simulink model "bh_wheel_dynamics_COMPARE_hand_SEME_to_MEME"  (R2019a)
settings: Solver=ode15s  StartTime=0.0  StopTime=80  FixedStep=0.001  RelTol=1e-6  EnableMultiTasking=on
undefined symbols (not defined in the file or in its folder): Ic_xx_val, sigbuilder_block
libraries: simulink_extras x6
settings Model: Creator=bhorton  LastModifiedBy=bhorton
settings SolverCC: ZeroCrossAlgorithm=Adaptive
settings DataIOCC: SaveOutput=off  SignalLogging=off  DSMLogging=off  VisualizeSimOutput=off  SaveTime=off  ReturnWorkspaceOutputs=off
settings OptimizationCC: LifeSpan=inf
settings DebuggingCC: AllowSymbolicDim=off  SFUnexpectedBacktrackingDiag=warning  SFNoUnconditionalDefaultTransitionDiag=warning  SFExecutionAtInitializationDiag=none  ArithmeticOperatorsInVariantConditions=warning
settings ModelReferenceCC: PropagateSignalLabelsOutOfModel=off
settings SFSimCC: SimUseLocalCustomCode=off
settings RTWCC: RTWUseLocalCustomCode=off
settings CodeAppCC: StateflowObjectComments=on
settings GRTTargetCC: TargetLangStandard=C89/C90 (ANSI)
settings ConfigComp: CovMetricSettings=dw  CovHtmlReporting=on  CovSaveCumulativeToWorkspaceVar=on  CovSaveSingleToWorkspaceVar=on  CovExternalEMLEnable=off
settings SimscapeCC: SimscapeNormalizeSystem=off

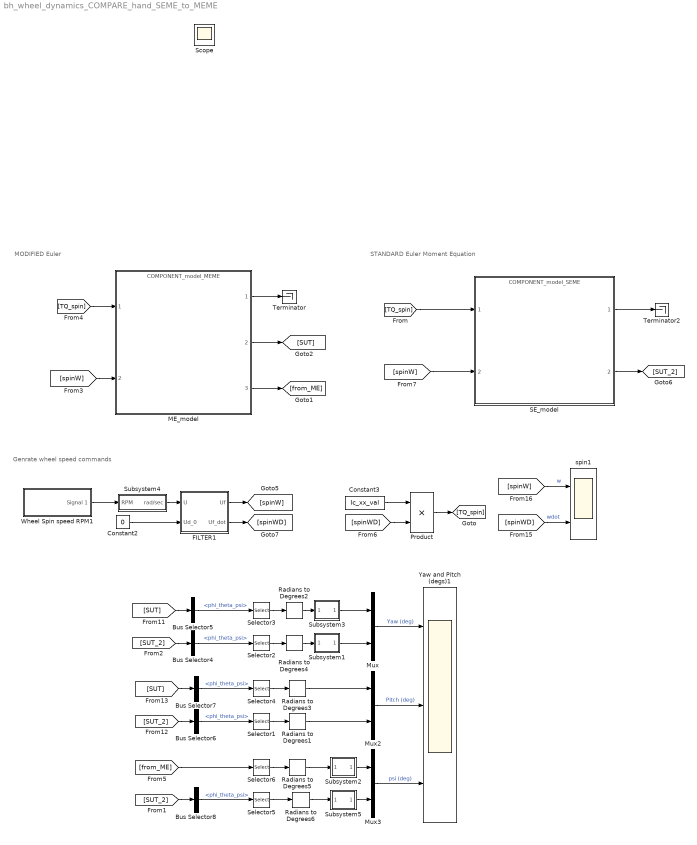
== system bh_wheel_dynamics_COMPARE_hand_SEME_to_MEME ==
  note: MODIFIED Euler
  note: STANDARD Euler Moment Equation
  note: Genrate wheel speed commands
  Bus Selector{4..8} (5 alike) : BusSelector  OutputSignals=phi_theta_psi
  Constant2 : Constant  Value=0
  Constant3 : Constant  Value=Ic_xx_val
  FILTER1 : Subsystem
  ME_model : ModelReference  ModelNameDialog=COMPONENT_model_MEME.slx  SimulationMode=Normal  ModelReferenceVersion=1.567
  Mux : Mux  Inputs=2
  Mux2 : Mux  Inputs=2
  Mux3 : Mux  Inputs=2
  Product : Product
  Radians to Degrees{1..6} (6 alike) : simulink_extras/Transformations/Radians to Degrees
  SE_model : ModelReference  ModelNameDialog=COMPONENT_model_SEME.slx  SimulationMode=Normal  ModelReferenceVersion=1.562
  Selector1 : Selector  InputPortWidth=3  IndexOptions=Index vector (dialog)  Indices=2  OutputSizes=1
  Selector2 : Selector  InputPortWidth=3  IndexOptions=Index vector (dialog)  Indices=1  OutputSizes=1
  Selector3 : Selector  InputPortWidth=3  IndexOptions=Index vector (dialog)  Indices=1  OutputSizes=1
  Selector4 : Selector  InputPortWidth=3  IndexOptions=Index vector (dialog)  Indices=2  OutputSizes=1
  Selector5 : Selector  InputPortWidth=3  IndexOptions=Index vector (dialog)  Indices=3  OutputSizes=1
  Selector6 : Selector  InputPortWidth=2  IndexOptions=Index vector (dialog)  Indices=2  OutputSizes=1
  Subsystem1 : Subsystem
      mask Display: disp(sprintf('Mod\n360'))
  Subsystem2 : Subsystem
      mask Display: disp(sprintf('Mod\n360'))
  Subsystem3 : Subsystem
      mask Display: disp(sprintf('Mod\n360'))
  Subsystem4 : Subsystem
  Subsystem5 : Subsystem
      mask Display: disp(sprintf('Mod\n360'))
  Terminator : Terminator
  Terminator2 : Terminator
  Wheel Spin speed RPM1 : Subsystem  Tag=STV Subsys  LoadFcn=sigbuilder_block('load');  StartFcn=sigbuilder_block('start');  StopFcn=sigbuilder_block('stop');  ClipboardFcn=sigbuilder_block('clipboard');  mask(Sigbuilder block){tuvar=[0:10]}
      mask help: Simulink:masks:SigbuilderBlock_MD
      mask init:
      | if ~strcmp(get_param(bdroot(gcbh),'SimulationStatus'),'stopped') tuvar = sigbuilder_block('maskInit'); end
      settings: CopyFcn=sigbuilder_block('copy');  DeleteFcn=sigbuilder_block('delete');  ModelCloseFcn=sigbuilder_block('modelClose');  PreSaveFcn=sigbuilder_block('preSave');  PauseFcn=sigbuilder_block('pause');  ContinueFcn=sigbuilder_block('continue');  NameChangeFcn=sigbuilder_block('namechange');  OpenFcn=sigbuilder_block('open',[6 6 1428 740.25 ]);  CloseFcn=sigbuilder_block('close');
      mask Display: plot(0, 0, 100, 100,[2, 2, 32, 32, 2], [68, 8, 8, 68, 68],[32, 2], [38, 38], [32, 19, 2],[53, 60, 44], [32, 17, 17, 2],[16, 16, 31, 31]);txt = getActiveGroup(gcbh);text(2, 100, txt,'verticalAlignment', 'top');
  Yaw and Pitch (degs)1 : Scope  NumInputPorts=3
  spin1 : Scope  NumInputPorts=2
  Scope : Scope
  wires:
  Selector1/1 -> Radians to Degrees1/1
  Radians to Degrees4/1 -> Subsystem1/1(In1)
  Radians to Degrees1/1 -> Mux2/2
  Selector2/1 -> Radians to Degrees4/1
  [SUT_2] -> Bus Selector6/1
  [SUT_2] -> Bus Selector4/1
  Bus Selector5/1 -> Selector3/1  "<phi_theta_psi>"
  Radians to Degrees2/1 -> Subsystem3/1(In1)
  Selector4/1 -> Radians to Degrees3/1
  Mux2/1 -> Yaw and Pitch (degs)1/2  "Pitch (deg)"
  Subsystem1/1(Out1) -> Mux/2
  [SUT] -> Bus Selector7/1
  Subsystem3/1(Out1) -> Mux/1
  Mux/1 -> Yaw and Pitch (degs)1/1  "Yaw (deg)"
  Bus Selector7/1 -> Selector4/1  "<phi_theta_psi>"
  Radians to Degrees3/1 -> Mux2/1
  Selector3/1 -> Radians to Degrees2/1
  Bus Selector6/1 -> Selector1/1  "<phi_theta_psi>"
  Bus Selector4/1 -> Selector2/1  "<phi_theta_psi>"
  [SUT] -> Bus Selector5/1
  Mux3/1 -> Yaw and Pitch (degs)1/3  "psi (deg)"
  [SUT_2] -> Bus Selector8/1
  Bus Selector8/1 -> Selector5/1  "<phi_theta_psi>"
  Selector5/1 -> Radians to Degrees6/1
  Selector6/1 -> Radians to Degrees5/1
  ME_model/2 -> [SUT]
  [TQ_spin] -> ME_model/1
  SE_model/2 -> [SUT_2]
  [spinW] -> SE_model/2
  [TQ_spin] -> SE_model/1
  SE_model/1 -> Terminator2/1
  ME_model/1 -> Terminator/1
  [spinW] -> ME_model/2
  FILTER1/2(Uf_dot) -> [spinWD]
  [spinWD] -> Product/2
  Wheel Spin speed RPM1/1(Signal 1) -> Subsystem4/1(RPM)
  Constant3/1 -> Product/1
  Constant2/1 -> FILTER1/2(Ud_0)
  FILTER1/1(Uf) -> [spinW]
  Subsystem4/1(rad/sec) -> FILTER1/1(U)
  [spinWD] -> spin1/2  "wdot"
  [spinW] -> spin1/1  "w"
  Product/1 -> [TQ_spin]
  ME_model/3 -> [from_ME]
  [from_ME] -> Selector6/1
  Radians to Degrees5/1 -> Subsystem2/1(In1)
  Radians to Degrees6/1 -> Subsystem5/1(In1)
  Subsystem2/1(Out1) -> Mux3/1
  Subsystem5/1(Out1) -> Mux3/2

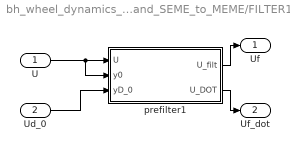
== system bh_wheel_dynamics_COMPARE_hand_SEME_to_MEME/FILTER1 ==
  U : Inport
  Ud_0 : Inport  Port=2
  prefilter1 : Subsystem  mask(Derivative Estimation){wn=2*pi*5, p=1}
      mask prompts: wn "Natural frequency, wn (rad/sec)"; p "Damping ratio, p"
      mask help:
      | A simple derivative estimator using a 2nd order representation between input and output.
      |
      | The integrators use a discrete FORWARd Euler rule, and a sample time needs to be specified.
      mask init:
      | str1 = sprintf('wn = %.2f', wn);
      | str2 = sprintf('p  = %.2f', p);
      | %str3 = sprintf('dt = %.2f', dt);
      | %str = char(str1,str2,str3);
      | %str3 = sprintf('dt = %.2f', dt);
      | str = char(str1,str2);
      mask Display: disp(str)
  Uf : Outport
  Uf_dot : Outport  Port=2
  wires:
  Ud_0/1 -> prefilter1/3(yD_0)
  prefilter1/2(U_DOT) -> Uf_dot/1
  prefilter1/1(U_filt) -> Uf/1
  U/1 -> prefilter1/2(y0), prefilter1/1(U)

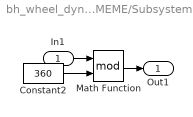
== system bh_wheel_dynamics_COMPARE_hand_SEME_to_MEME/Subsystem1 ==
  In1 : Inport
  Constant2 : Constant  Value=360
  Math Function : Math  Operator=mod  SaturateOnIntegerOverflow=on
  Out1 : Outport
  wires:
  Math Function/1 -> Out1/1
  In1/1 -> Math Function/1
  Constant2/1 -> Math Function/2

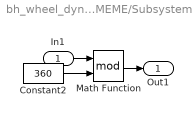
== system bh_wheel_dynamics_COMPARE_hand_SEME_to_MEME/Subsystem2 ==
  In1 : Inport
  Constant2 : Constant  Value=360
  Math Function : Math  Operator=mod  SaturateOnIntegerOverflow=on
  Out1 : Outport
  wires:
  Math Function/1 -> Out1/1
  In1/1 -> Math Function/1
  Constant2/1 -> Math Function/2

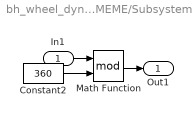
== system bh_wheel_dynamics_COMPARE_hand_SEME_to_MEME/Subsystem3 ==
  In1 : Inport
  Constant2 : Constant  Value=360
  Math Function : Math  Operator=mod  SaturateOnIntegerOverflow=on
  Out1 : Outport
  wires:
  Math Function/1 -> Out1/1
  In1/1 -> Math Function/1
  Constant2/1 -> Math Function/2

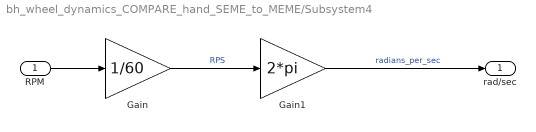
== system bh_wheel_dynamics_COMPARE_hand_SEME_to_MEME/Subsystem4 ==
  RPM : Inport
  Gain : Gain  Gain=1/60
  Gain1 : Gain  Gain=2*pi
  rad/sec : Outport
  wires:
  RPM/1 -> Gain/1
  Gain/1 -> Gain1/1  "RPS"
  Gain1/1 -> rad/sec/1  "radians_per_sec"

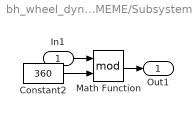
== system bh_wheel_dynamics_COMPARE_hand_SEME_to_MEME/Subsystem5 ==
  In1 : Inport
  Constant2 : Constant  Value=360
  Math Function : Math  Operator=mod  SaturateOnIntegerOverflow=on
  Out1 : Outport
  wires:
  Math Function/1 -> Out1/1
  In1/1 -> Math Function/1
  Constant2/1 -> Math Function/2

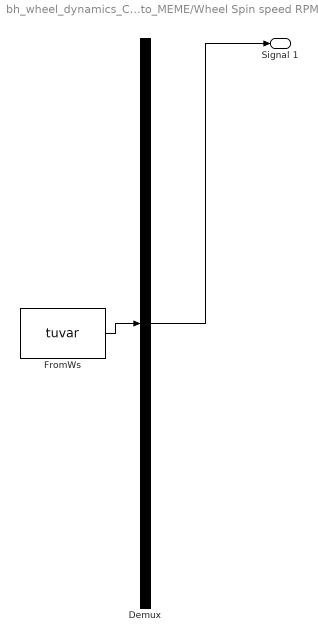
== system bh_wheel_dynamics_COMPARE_hand_SEME_to_MEME/Wheel Spin speed RPM1 ==
  Demux : Demux  Tag=STV Demux  Outputs=1
  FromWs : FromWorkspace  Tag=STV FromWs  VariableName=tuvar  SampleTime=0
      SigBuilderData=|
      | common.afterFinalStr = 'Extrapolate'
      | common.sampleTime = 0
      | dataSet(1).timeRange = [0 60]
      | dataSet(1).name = 'RAMP_DOWN'
      | dataSet(2).timeRange = [0 80]
      | dataSet(2).name = 'STAIRCASE_DOWN'
      | dataSet(3).timeRange = [0 60]
      | dataSet(3).name = 'STAIRCASE_UP'
      | sbobj.Groups(1).Name = 'RAMP_DOWN'
      | sbobj.Groups(1).Signals.Name = 'Signal 1'
      | sbobj.Groups(1).Signals.XData = [0 60]
      | sbobj.Groups(1).Signals.YData = [2000 0]
      | sbobj.Groups(1).TimeRange = [0 60]
      | sbobj.Groups(2).Name = 'STAIRCASE_DOWN'
      | sbobj.Groups(2).Signals.Name = 'Signal 1'
      | sbobj.Groups(2).Signals.XData = [0 10.1 10.1 20 20 30 30 39.9 39.9 49.9 49.9 60.2 60.2 70 70 80]
      | sbobj.Groups(2).Signals.YData = [2000 2000 1500 1500 1000 1000 750 750 500 500 150 150 60 60 0 0]
      | sbobj.Groups(2).TimeRange = [0 80]
      | sbobj.Groups(3).Name = 'STAIRCASE_UP'
      | sbobj.Groups(3).Signals.Name = 'Signal 1'
      | sbobj.Groups(3).Signals.XData = [0 9.9 9.9 19.9 19.9 30.1 30.1 39.9 39.9 49.9 49.9 60]
      | sbobj.Groups(3).Signals.YData = [2000 2000 2200 2200 2400 2400 2610 2610 1800 1800 1600 1600]
      | sbobj.Groups(3).TimeRange = [0 60]
  Signal 1 : Outport  Tag=STV Outport
  wires:
  Demux/1 -> Signal 1/1
  FromWs/1 -> Demux/1

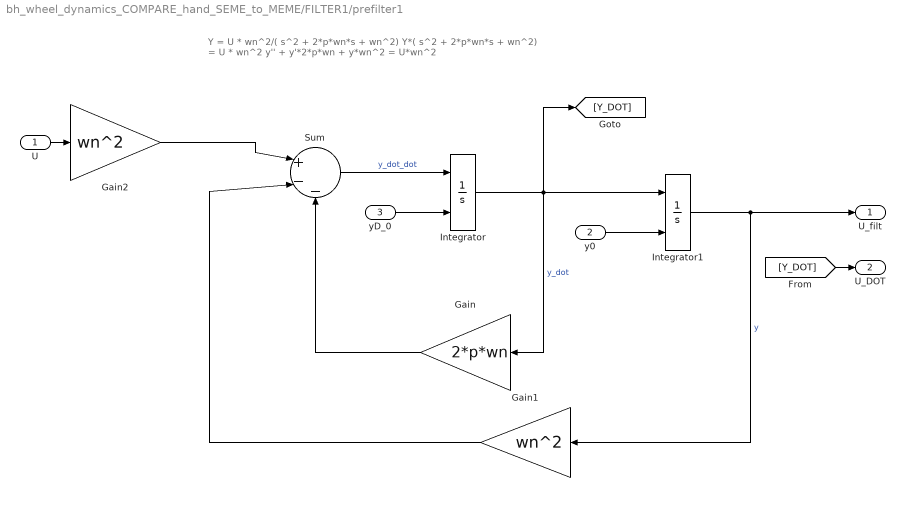
== system bh_wheel_dynamics_COMPARE_hand_SEME_to_MEME/FILTER1/prefilter1 ==
  note: Y = U *     wn^2/( s^2 + 2*p*wn*s + wn^2)
      | Y*( s^2 + 2*p*wn*s + wn^2) = U * wn^2
      |
      | y'' + y'*2*p*wn + y*wn^2 = U*wn^2
  U : Inport
  y0 : Inport  Port=2
  yD_0 : Inport  Port=3
  Gain : Gain  Gain=2*p*wn
  Gain1 : Gain  Gain=wn^2
  Gain2 : Gain  Gain=wn^2
  Integrator : Integrator  InitialConditionSource=external
  Integrator1 : Integrator  InitialConditionSource=external
  Sum : Sum  Inputs=|+--
  U_filt : Outport
  U_DOT : Outport  Port=2
  wires:
  Integrator/1 -> [Y_DOT], Gain/1, Integrator1/1  "y_dot"
  Sum/1 -> Integrator/1  "y_dot_dot"
  Integrator1/1 -> Gain1/1, U_filt/1  "y"
  U/1 -> Gain2/1
  Gain2/1 -> Sum/1
  Gain/1 -> Sum/3
  Gain1/1 -> Sum/2
  [Y_DOT] -> U_DOT/1
  yD_0/1 -> Integrator/2
  y0/1 -> Integrator1/2
